simulink model "Relu_NoOutFB_4_4_1_HW_C6"  (R2012b)
settings: Solver=FixedStepDiscrete  SolverMode=SingleTasking  StartTime=0.0  StopTime=limSim  FixedStep=ts  RelTol=1e-3
undefined symbols (not defined in the file): alpha, delayMulx, delayMuly, delayROMSig, M2, M3, mu, ts
libraries: xbsIndex_r4 x1578, roblocks x1
(part 1 of 13)
settings Model: Creator=Marcelo  LastModifiedBy=snata
settings DataIOCC: SignalLoggingSaveFormat=ModelDataLogs
settings DebuggingCC: MultiTaskDSMMsg=warning  MultiTaskCondExecSysMsg=none  FcnCallInpInsideContextMsg=UseLocalSettings  StrictBusMsg=None
settings RTWCC: IncludeERTFirstTime=on
settings CodeAppCC: CustomSymbolStrType=$N$R$M_T  InternalIdentifier=Shortened
settings GRTTargetCC: CombineOutputUpdateFcns=off  GRTInterface=on

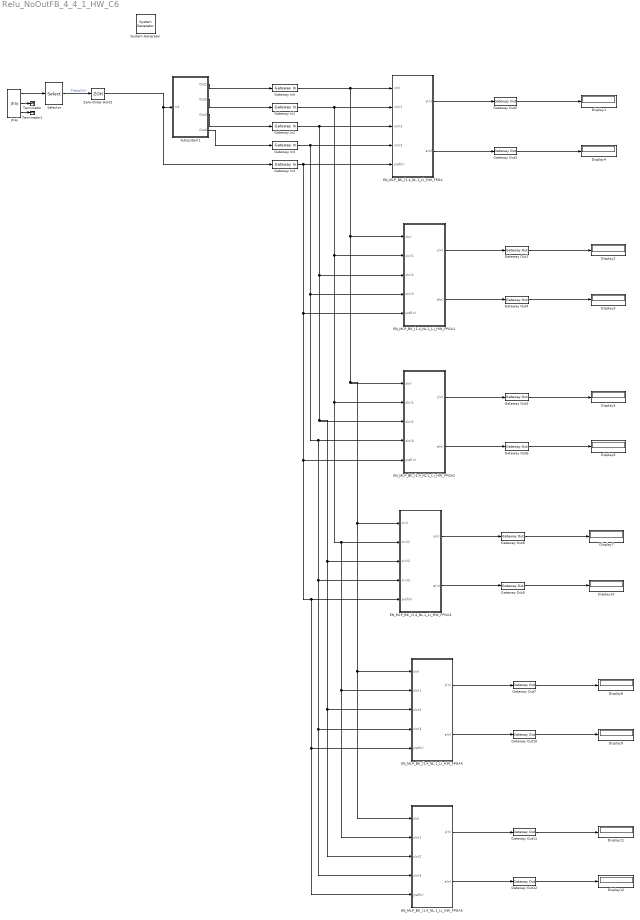
== system Relu_NoOutFB_4_4_1_HW_C6 ==
  " System Generator" : xbsIndex_r4/ System Generator  Tag=genX  xilinxfamily=virtex6  part=xc6vlx240t  speed=-1  package=ff1156  synthesis_tool=XST  clock_wrapper=Clock Enables  directory=C:/Users/snata/Documents/Netlists/RELU_SemReal_18_14  proj_type=Project Navigator  Synth_file=XST Defaults  Impl_file=ISE Defaults  testbench=off  simulink_period=0.01  sysclk_period=10  dcm_input_clock_period=10  incr_netlist=off  trim_vbits=Everywhere in SubSystem  dbl_ovrd=According to Block Masks  core_generation=According to Block Masks  run_coregen=off  deprecated_control=off  eval_field=0  block_type=sysgen
  Display{1..12} (12 alike) : Display
  EN_MLP_BK_(1,4_NL,1_L)_HW_FPGA : Subsystem
  EN_MLP_BK_(1,4_NL,1_L)_HW_FPGA1 : Subsystem
  EN_MLP_BK_(1,4_NL,1_L)_HW_FPGA2 : Subsystem
  EN_MLP_BK_(1,4_NL,1_L)_HW_FPGA3 : Subsystem
  EN_MLP_BK_(1,4_NL,1_L)_HW_FPGA4 : Subsystem
  EN_MLP_BK_(1,4_NL,1_L)_HW_FPGA5 : Subsystem
  Gateway In{1..5} (5 alike) : xbsIndex_r4/Gateway In  gui_display_data_type=Fixed-point  arith_type="Signed  (2's comp)"  n_bits=nb  bin_pt=bp  preci_type=Single  exp_width=8  frac_width=24  quantization="Round  (unbiased: +/- Inf)"  overflow=Saturate  period=ts  dbl_ovrd=off  timing_constraint=None  locs_specified=off  LOCs={}  UseAsADC=off  ADCChannel='1'  inherit_from_input=off  hdl_port=on  block_type=gatewayin
  Gateway Out{1..12} (12 alike) : xbsIndex_r4/Gateway Out  inherit_from_input=off  hdl_port=on  timing_constraint=None  locs_specified=off  LOCs={}  UseAsDAC=off  DACChannel='1'  block_type=gatewayout
      settings: infoedit="Gateway out block.  Converts Xilinx fixed point inputs into ouputs of type Simulink integer, double, or fixed point.<br><br>Hardware notes:  In hardware these blocks become top level output ports or are discarded, depending on how they are configured."
  Selector : Selector  InputPortWidth=3  IndexOptions=Index vector (dialog)  Indices=[1]  OutputSizes=1
  Subsystem1 : Subsystem
  Terminator : Terminator
  Terminator1 : Terminator
  Zero-Order Hold1 : ZeroOrderHold  SampleTime=ts
  jtraj : roblocks/Trajectory/jtraj  q0=[0 -pi/2 pi]  qf=[pi/2 pi/4 pi/2]  tmax=limSim  ts=ts
  wires:
  jtraj/1 -> Selector/1
  Subsystem1/1(Out1) -> Gateway In5/1
  Subsystem1/2(Out2) -> Gateway In1/1
  Subsystem1/3(Out3) -> Gateway In2/1
  Selector/1 -> Zero-Order Hold1/1  "Theta1(n)"
  Subsystem1/4(Out4) -> Gateway In3/1
  Zero-Order Hold1/1 -> Subsystem1/1(In1), Gateway In4/1
  jtraj/2 -> Terminator/1
  jtraj/3 -> Terminator1/1
  EN_MLP_BK_(1,4_NL,1_L)_HW_FPGA/2(e(n)) -> Gateway Out3/1
  Gateway Out3/1 -> Display4/1
  Gateway Out2/1 -> Display1/1
  EN_MLP_BK_(1,4_NL,1_L)_HW_FPGA/1(y(n)) -> Gateway Out2/1
  EN_MLP_BK_(1,4_NL,1_L)_HW_FPGA1/2(e(n)) -> Gateway Out4/1
  EN_MLP_BK_(1,4_NL,1_L)_HW_FPGA1/1(y(n)) -> Gateway Out1/1
  Gateway Out4/1 -> Display3/1
  Gateway Out1/1 -> Display2/1
  EN_MLP_BK_(1,4_NL,1_L)_HW_FPGA2/2(e(n)) -> Gateway Out6/1
  EN_MLP_BK_(1,4_NL,1_L)_HW_FPGA2/1(y(n)) -> Gateway Out5/1
  Gateway Out6/1 -> Display6/1
  Gateway Out5/1 -> Display5/1
  EN_MLP_BK_(1,4_NL,1_L)_HW_FPGA3/2(e(n)) -> Gateway Out9/1
  Gateway Out9/1 -> Display10/1
  Gateway Out8/1 -> Display7/1
  EN_MLP_BK_(1,4_NL,1_L)_HW_FPGA3/1(y(n)) -> Gateway Out8/1
  EN_MLP_BK_(1,4_NL,1_L)_HW_FPGA4/2(e(n)) -> Gateway Out10/1
  EN_MLP_BK_(1,4_NL,1_L)_HW_FPGA4/1(y(n)) -> Gateway Out7/1
  Gateway Out10/1 -> Display9/1
  Gateway Out7/1 -> Display8/1
  EN_MLP_BK_(1,4_NL,1_L)_HW_FPGA5/2(e(n)) -> Gateway Out12/1
  Gateway In5/1 -> EN_MLP_BK_(1,4_NL,1_L)_HW_FPGA3/1(x(n)), EN_MLP_BK_(1,4_NL,1_L)_HW_FPGA4/1(x(n)), EN_MLP_BK_(1,4_NL,1_L)_HW_FPGA5/1(x(n)), EN_MLP_BK_(1,4_NL,1_L)_HW_FPGA2/1(x(n)), EN_MLP_BK_(1,4_NL,1_L)_HW_FPGA1/1(x(n)), EN_MLP_BK_(1,4_NL,1_L)_HW_FPGA/1(x(n))
  Gateway In4/1 -> EN_MLP_BK_(1,4_NL,1_L)_HW_FPGA3/5(yref(n)), EN_MLP_BK_(1,4_NL,1_L)_HW_FPGA4/5(yref(n)), EN_MLP_BK_(1,4_NL,1_L)_HW_FPGA5/5(yref(n)), EN_MLP_BK_(1,4_NL,1_L)_HW_FPGA2/5(yref(n)), EN_MLP_BK_(1,4_NL,1_L)_HW_FPGA1/5(yref(n)), EN_MLP_BK_(1,4_NL,1_L)_HW_FPGA/5(yref(n))
  Gateway In1/1 -> EN_MLP_BK_(1,4_NL,1_L)_HW_FPGA3/2(x(n)1), EN_MLP_BK_(1,4_NL,1_L)_HW_FPGA4/2(x(n)1), EN_MLP_BK_(1,4_NL,1_L)_HW_FPGA5/2(x(n)1), EN_MLP_BK_(1,4_NL,1_L)_HW_FPGA2/2(x(n)1), EN_MLP_BK_(1,4_NL,1_L)_HW_FPGA1/2(x(n)1), EN_MLP_BK_(1,4_NL,1_L)_HW_FPGA/2(x(n)1)
  Gateway In2/1 -> EN_MLP_BK_(1,4_NL,1_L)_HW_FPGA3/3(x(n)2), EN_MLP_BK_(1,4_NL,1_L)_HW_FPGA4/3(x(n)2), EN_MLP_BK_(1,4_NL,1_L)_HW_FPGA5/3(x(n)2), EN_MLP_BK_(1,4_NL,1_L)_HW_FPGA2/3(x(n)2), EN_MLP_BK_(1,4_NL,1_L)_HW_FPGA1/3(x(n)2), EN_MLP_BK_(1,4_NL,1_L)_HW_FPGA/3(x(n)2)
  EN_MLP_BK_(1,4_NL,1_L)_HW_FPGA5/1(y(n)) -> Gateway Out11/1
  Gateway In3/1 -> EN_MLP_BK_(1,4_NL,1_L)_HW_FPGA3/4(x(n)3), EN_MLP_BK_(1,4_NL,1_L)_HW_FPGA4/4(x(n)3), EN_MLP_BK_(1,4_NL,1_L)_HW_FPGA5/4(x(n)3), EN_MLP_BK_(1,4_NL,1_L)_HW_FPGA2/4(x(n)3), EN_MLP_BK_(1,4_NL,1_L)_HW_FPGA1/4(x(n)3), EN_MLP_BK_(1,4_NL,1_L)_HW_FPGA/4(x(n)3)
  Gateway Out12/1 -> Display12/1
  Gateway Out11/1 -> Display11/1

== system Relu_NoOutFB_4_4_1_HW_C6/EN_MLP_BK_(1,4_NL,1_L)_HW_FPGA ==
  x(n) : Inport
  x(n)1 : Inport  Port=2
  x(n)2 : Inport  Port=3
  x(n)3 : Inport  Port=4
  yref(n) : Inport  Port=5
  MLP_BK_(2,4_NL,1_L)_HW_FPGA : Subsystem
  y(n) : Outport
  e(n) : Outport  Port=2
  wires:
  yref(n)/1 -> MLP_BK_(2,4_NL,1_L)_HW_FPGA/5(y_ref(n))
  x(n)/1 -> MLP_BK_(2,4_NL,1_L)_HW_FPGA/1(x_1(n))  "x(n)"
  MLP_BK_(2,4_NL,1_L)_HW_FPGA/2(e(n)) -> e(n)/1
  x(n)1/1 -> MLP_BK_(2,4_NL,1_L)_HW_FPGA/2(x_2(n))
  x(n)2/1 -> MLP_BK_(2,4_NL,1_L)_HW_FPGA/3(x_3(n))
  MLP_BK_(2,4_NL,1_L)_HW_FPGA/1(y(n)) -> y(n)/1
  x(n)3/1 -> MLP_BK_(2,4_NL,1_L)_HW_FPGA/4(x_4(n))

== system Relu_NoOutFB_4_4_1_HW_C6/EN_MLP_BK_(1,4_NL,1_L)_HW_FPGA1 ==
  x(n) : Inport
  x(n)1 : Inport  Port=2
  x(n)2 : Inport  Port=3
  x(n)3 : Inport  Port=4
  yref(n) : Inport  Port=5
  MLP_BK_(2,4_NL,1_L)_HW_FPGA : Subsystem
  y(n) : Outport
  e(n) : Outport  Port=2
  wires:
  x(n)3/1 -> MLP_BK_(2,4_NL,1_L)_HW_FPGA/4(x_4(n))
  MLP_BK_(2,4_NL,1_L)_HW_FPGA/1(y(n)) -> y(n)/1
  x(n)2/1 -> MLP_BK_(2,4_NL,1_L)_HW_FPGA/3(x_3(n))
  x(n)1/1 -> MLP_BK_(2,4_NL,1_L)_HW_FPGA/2(x_2(n))
  MLP_BK_(2,4_NL,1_L)_HW_FPGA/2(e(n)) -> e(n)/1
  x(n)/1 -> MLP_BK_(2,4_NL,1_L)_HW_FPGA/1(x_1(n))  "x(n)"
  yref(n)/1 -> MLP_BK_(2,4_NL,1_L)_HW_FPGA/5(y_ref(n))

== system Relu_NoOutFB_4_4_1_HW_C6/EN_MLP_BK_(1,4_NL,1_L)_HW_FPGA2 ==
  x(n) : Inport
  x(n)1 : Inport  Port=2
  x(n)2 : Inport  Port=3
  x(n)3 : Inport  Port=4
  yref(n) : Inport  Port=5
  MLP_BK_(2,4_NL,1_L)_HW_FPGA : Subsystem
  y(n) : Outport
  e(n) : Outport  Port=2
  wires:
  yref(n)/1 -> MLP_BK_(2,4_NL,1_L)_HW_FPGA/5(y_ref(n))
  x(n)/1 -> MLP_BK_(2,4_NL,1_L)_HW_FPGA/1(x_1(n))  "x(n)"
  MLP_BK_(2,4_NL,1_L)_HW_FPGA/2(e(n)) -> e(n)/1
  x(n)1/1 -> MLP_BK_(2,4_NL,1_L)_HW_FPGA/2(x_2(n))
  x(n)2/1 -> MLP_BK_(2,4_NL,1_L)_HW_FPGA/3(x_3(n))
  MLP_BK_(2,4_NL,1_L)_HW_FPGA/1(y(n)) -> y(n)/1
  x(n)3/1 -> MLP_BK_(2,4_NL,1_L)_HW_FPGA/4(x_4(n))

== system Relu_NoOutFB_4_4_1_HW_C6/EN_MLP_BK_(1,4_NL,1_L)_HW_FPGA3 ==
  x(n) : Inport
  x(n)1 : Inport  Port=2
  x(n)2 : Inport  Port=3
  x(n)3 : Inport  Port=4
  yref(n) : Inport  Port=5
  MLP_BK_(2,4_NL,1_L)_HW_FPGA : Subsystem
  y(n) : Outport
  e(n) : Outport  Port=2
  wires:
  x(n)3/1 -> MLP_BK_(2,4_NL,1_L)_HW_FPGA/4(x_4(n))
  MLP_BK_(2,4_NL,1_L)_HW_FPGA/1(y(n)) -> y(n)/1
  x(n)2/1 -> MLP_BK_(2,4_NL,1_L)_HW_FPGA/3(x_3(n))
  x(n)1/1 -> MLP_BK_(2,4_NL,1_L)_HW_FPGA/2(x_2(n))
  MLP_BK_(2,4_NL,1_L)_HW_FPGA/2(e(n)) -> e(n)/1
  x(n)/1 -> MLP_BK_(2,4_NL,1_L)_HW_FPGA/1(x_1(n))  "x(n)"
  yref(n)/1 -> MLP_BK_(2,4_NL,1_L)_HW_FPGA/5(y_ref(n))

== system Relu_NoOutFB_4_4_1_HW_C6/EN_MLP_BK_(1,4_NL,1_L)_HW_FPGA4 ==
  x(n) : Inport
  x(n)1 : Inport  Port=2
  x(n)2 : Inport  Port=3
  x(n)3 : Inport  Port=4
  yref(n) : Inport  Port=5
  MLP_BK_(2,4_NL,1_L)_HW_FPGA : Subsystem
  y(n) : Outport
  e(n) : Outport  Port=2
  wires:
  yref(n)/1 -> MLP_BK_(2,4_NL,1_L)_HW_FPGA/5(y_ref(n))
  x(n)/1 -> MLP_BK_(2,4_NL,1_L)_HW_FPGA/1(x_1(n))  "x(n)"
  MLP_BK_(2,4_NL,1_L)_HW_FPGA/2(e(n)) -> e(n)/1
  x(n)1/1 -> MLP_BK_(2,4_NL,1_L)_HW_FPGA/2(x_2(n))
  x(n)2/1 -> MLP_BK_(2,4_NL,1_L)_HW_FPGA/3(x_3(n))
  MLP_BK_(2,4_NL,1_L)_HW_FPGA/1(y(n)) -> y(n)/1
  x(n)3/1 -> MLP_BK_(2,4_NL,1_L)_HW_FPGA/4(x_4(n))

== system Relu_NoOutFB_4_4_1_HW_C6/EN_MLP_BK_(1,4_NL,1_L)_HW_FPGA5 ==
  x(n) : Inport
  x(n)1 : Inport  Port=2
  x(n)2 : Inport  Port=3
  x(n)3 : Inport  Port=4
  yref(n) : Inport  Port=5
  MLP_BK_(2,4_NL,1_L)_HW_FPGA : Subsystem
  y(n) : Outport
  e(n) : Outport  Port=2
  wires:
  x(n)3/1 -> MLP_BK_(2,4_NL,1_L)_HW_FPGA/4(x_4(n))
  MLP_BK_(2,4_NL,1_L)_HW_FPGA/1(y(n)) -> y(n)/1
  x(n)2/1 -> MLP_BK_(2,4_NL,1_L)_HW_FPGA/3(x_3(n))
  x(n)1/1 -> MLP_BK_(2,4_NL,1_L)_HW_FPGA/2(x_2(n))
  MLP_BK_(2,4_NL,1_L)_HW_FPGA/2(e(n)) -> e(n)/1
  x(n)/1 -> MLP_BK_(2,4_NL,1_L)_HW_FPGA/1(x_1(n))  "x(n)"
  yref(n)/1 -> MLP_BK_(2,4_NL,1_L)_HW_FPGA/5(y_ref(n))

== system Relu_NoOutFB_4_4_1_HW_C6/Subsystem1 ==
  In1 : Inport
  Delay{1..6} (6 alike) : Delay  DelayLength=1
  Terminator : Terminator
  Out1 : Outport
  Out2 : Outport  Port=2
  Out3 : Outport  Port=3
  Out4 : Outport  Port=4
  wires:
  Delay4/1 -> Delay1/1, Out3/1
  Delay2/1 -> Out2/1, Delay4/1
  Delay3/1 -> Out1/1, Delay2/1
  In1/1 -> Delay3/1
  Delay1/1 -> Out4/1, Delay5/1
  Delay5/1 -> Delay6/1
  Delay6/1 -> Terminator/1

== system Relu_NoOutFB_4_4_1_HW_C6/EN_MLP_BK_(1,4_NL,1_L)_HW_FPGA/MLP_BK_(2,4_NL,1_L)_HW_FPGA ==
  x_1(n) : Inport
  x_2(n) : Inport  Port=2
  x_3(n) : Inport  Port=3
  x_4(n) : Inport  Port=4
  y_ref(n) : Inport  Port=5
  AddSub : xbsIndex_r4/AddSub  mode=Subtraction  use_carryin=off  use_carryout=off  en=off  latency=0  precision=User Defined  arith_type="Signed  (2's comp)"  n_bits=nb  bin_pt=bp  quantization="Round  (unbiased: +/- Inf)"  overflow=Wrap  dbl_ovrd=off  use_behavioral_HDL=off  hw_selection=Fabric  pipelined=off  block_type=addsub
  BK (2,4_NL,1_L) : Subsystem
  Delay{,1..4} (5 alike) : xbsIndex_r4/Delay  rst=off  infoeditControl=Selection of Reset will increase slice count due to use of real FFs and instead of SRLs  en=off  latency=delayROMSig+delayMulx+delayMuly  dbl_ovrd=off  reg_retiming=off  block_type=delay
  MLP (2,4_NL,1_L) : Subsystem
  y(n) : Outport
  e(n) : Outport  Port=2
  wires:
  Delay/1 -> AddSub/1
  y_ref(n)/1 -> Delay/1
  x_1(n)/1 -> MLP (2,4_NL,1_L)/4(x_1(n))
  BK (2,4_NL,1_L)/1(Wy_10(n)) -> MLP (2,4_NL,1_L)/29(Wy_10(n))
  AddSub/1 -> e(n)/1, BK (2,4_NL,1_L)/11(e(n))
  BK (2,4_NL,1_L)/2(Wy_11(n)) -> MLP (2,4_NL,1_L)/28(Wy_11(n))
  x_2(n)/1 -> MLP (2,4_NL,1_L)/3(x_2(n))
  x_3(n)/1 -> MLP (2,4_NL,1_L)/2(x_3(n))
  x_4(n)/1 -> MLP (2,4_NL,1_L)/1(x_4(n))
  BK (2,4_NL,1_L)/3(Wy_12(n)) -> MLP (2,4_NL,1_L)/27(Wy_12(n))
  BK (2,4_NL,1_L)/4(Wy_13(n)) -> MLP (2,4_NL,1_L)/26(Wy_13(n))
  BK (2,4_NL,1_L)/5(Wy_14(n)) -> MLP (2,4_NL,1_L)/25(Wy_14(n))
  BK (2,4_NL,1_L)/6(Wx_10(n)) -> MLP (2,4_NL,1_L)/24(Wx_10(n))
  BK (2,4_NL,1_L)/7(Wx_11(n)) -> MLP (2,4_NL,1_L)/23(Wx_11(n))
  BK (2,4_NL,1_L)/8(Wx_12(n)) -> MLP (2,4_NL,1_L)/22(Wx_12(n))
  BK (2,4_NL,1_L)/9(Wx_13(n)) -> MLP (2,4_NL,1_L)/21(Wx_13(n))
  BK (2,4_NL,1_L)/10(Wx_14(n)) -> MLP (2,4_NL,1_L)/20(Wx_14(n))
  BK (2,4_NL,1_L)/11(Wx_20(n)) -> MLP (2,4_NL,1_L)/19(Wx_20(n))
  BK (2,4_NL,1_L)/12(Wx_21(n)) -> MLP (2,4_NL,1_L)/18(Wx_21(n))
  BK (2,4_NL,1_L)/13(Wx_22(n)) -> MLP (2,4_NL,1_L)/17(Wx_22(n))
  BK (2,4_NL,1_L)/14(Wx_23(n)) -> MLP (2,4_NL,1_L)/16(Wx_23(n))
  BK (2,4_NL,1_L)/15(Wx_24(n)) -> MLP (2,4_NL,1_L)/15(Wx_24(n))
  BK (2,4_NL,1_L)/16(Wx_30(n)) -> MLP (2,4_NL,1_L)/14(Wx_30(n))
  BK (2,4_NL,1_L)/17(Wx_31(n)) -> MLP (2,4_NL,1_L)/13(Wx_31(n))
  BK (2,4_NL,1_L)/18(Wx_32(n)) -> MLP (2,4_NL,1_L)/12(Wx_32(n)1)
  BK (2,4_NL,1_L)/19(Wx_33(n)) -> MLP (2,4_NL,1_L)/11(Wx_33(n))
  BK (2,4_NL,1_L)/20(Wx_34(n)) -> MLP (2,4_NL,1_L)/10(Wx_34(n))
  BK (2,4_NL,1_L)/21(Wx_40(n)) -> MLP (2,4_NL,1_L)/9(Wx_40(n))
  BK (2,4_NL,1_L)/22(Wx_41(n)) -> MLP (2,4_NL,1_L)/8(Wx_41(n))
  BK (2,4_NL,1_L)/23(Wx_42(n)) -> MLP (2,4_NL,1_L)/7(Wx_42(n))
  BK (2,4_NL,1_L)/24(Wx_43(n)) -> MLP (2,4_NL,1_L)/6(Wx_43(n))
  BK (2,4_NL,1_L)/25(Wx_44(n)) -> MLP (2,4_NL,1_L)/5(Wx_44(n))
  MLP (2,4_NL,1_L)/11(x_4(n)bp) -> Delay1/1
  MLP (2,4_NL,1_L)/10(x_3(n)bp) -> Delay2/1
  MLP (2,4_NL,1_L)/9(x_2(n)bp) -> Delay3/1
  MLP (2,4_NL,1_L)/8(x_1(n)bp) -> Delay4/1
  MLP (2,4_NL,1_L)/6(z_4(n)) -> BK (2,4_NL,1_L)/6(z_4(n))
  MLP (2,4_NL,1_L)/5(z_3(n)) -> BK (2,4_NL,1_L)/7(z_3(n))
  MLP (2,4_NL,1_L)/4(z_2(n)) -> BK (2,4_NL,1_L)/8(z_2(n))
  MLP (2,4_NL,1_L)/3(z_1(n)) -> BK (2,4_NL,1_L)/9(z_1(n))
  MLP (2,4_NL,1_L)/2(z_0(n)) -> BK (2,4_NL,1_L)/10(z_0(n))
  MLP (2,4_NL,1_L)/1(y_0(n)) -> y(n)/1, AddSub/2
  Delay1/1 -> BK (2,4_NL,1_L)/1(x_4(n))
  Delay2/1 -> BK (2,4_NL,1_L)/2(x_3(n))
  Delay3/1 -> BK (2,4_NL,1_L)/3(x_2(n))
  Delay4/1 -> BK (2,4_NL,1_L)/4(x_1(n))
  MLP (2,4_NL,1_L)/7(x_0(n)bp) -> BK (2,4_NL,1_L)/5(x_0(n))

== system Relu_NoOutFB_4_4_1_HW_C6/EN_MLP_BK_(1,4_NL,1_L)_HW_FPGA1/MLP_BK_(2,4_NL,1_L)_HW_FPGA ==
  x_1(n) : Inport
  x_2(n) : Inport  Port=2
  x_3(n) : Inport  Port=3
  x_4(n) : Inport  Port=4
  y_ref(n) : Inport  Port=5
  AddSub : xbsIndex_r4/AddSub  mode=Subtraction  use_carryin=off  use_carryout=off  en=off  latency=0  precision=User Defined  arith_type="Signed  (2's comp)"  n_bits=nb  bin_pt=bp  quantization="Round  (unbiased: +/- Inf)"  overflow=Wrap  dbl_ovrd=off  use_behavioral_HDL=off  hw_selection=Fabric  pipelined=off  block_type=addsub
  BK (2,4_NL,1_L) : Subsystem
  Delay{,1..4} (5 alike) : xbsIndex_r4/Delay  rst=off  infoeditControl=Selection of Reset will increase slice count due to use of real FFs and instead of SRLs  en=off  latency=delayROMSig+delayMulx+delayMuly  dbl_ovrd=off  reg_retiming=off  block_type=delay
  MLP (2,4_NL,1_L) : Subsystem
  y(n) : Outport
  e(n) : Outport  Port=2
  wires:
  MLP (2,4_NL,1_L)/7(x_0(n)bp) -> BK (2,4_NL,1_L)/5(x_0(n))
  Delay4/1 -> BK (2,4_NL,1_L)/4(x_1(n))
  Delay3/1 -> BK (2,4_NL,1_L)/3(x_2(n))
  Delay2/1 -> BK (2,4_NL,1_L)/2(x_3(n))
  Delay1/1 -> BK (2,4_NL,1_L)/1(x_4(n))
  MLP (2,4_NL,1_L)/1(y_0(n)) -> AddSub/2, y(n)/1
  MLP (2,4_NL,1_L)/2(z_0(n)) -> BK (2,4_NL,1_L)/10(z_0(n))
  MLP (2,4_NL,1_L)/3(z_1(n)) -> BK (2,4_NL,1_L)/9(z_1(n))
  MLP (2,4_NL,1_L)/4(z_2(n)) -> BK (2,4_NL,1_L)/8(z_2(n))
  MLP (2,4_NL,1_L)/5(z_3(n)) -> BK (2,4_NL,1_L)/7(z_3(n))
  MLP (2,4_NL,1_L)/6(z_4(n)) -> BK (2,4_NL,1_L)/6(z_4(n))
  MLP (2,4_NL,1_L)/8(x_1(n)bp) -> Delay4/1
  MLP (2,4_NL,1_L)/9(x_2(n)bp) -> Delay3/1
  MLP (2,4_NL,1_L)/10(x_3(n)bp) -> Delay2/1
  MLP (2,4_NL,1_L)/11(x_4(n)bp) -> Delay1/1
  BK (2,4_NL,1_L)/25(Wx_44(n)) -> MLP (2,4_NL,1_L)/5(Wx_44(n))
  BK (2,4_NL,1_L)/24(Wx_43(n)) -> MLP (2,4_NL,1_L)/6(Wx_43(n))
  BK (2,4_NL,1_L)/23(Wx_42(n)) -> MLP (2,4_NL,1_L)/7(Wx_42(n))
  BK (2,4_NL,1_L)/22(Wx_41(n)) -> MLP (2,4_NL,1_L)/8(Wx_41(n))
  BK (2,4_NL,1_L)/21(Wx_40(n)) -> MLP (2,4_NL,1_L)/9(Wx_40(n))
  BK (2,4_NL,1_L)/20(Wx_34(n)) -> MLP (2,4_NL,1_L)/10(Wx_34(n))
  BK (2,4_NL,1_L)/19(Wx_33(n)) -> MLP (2,4_NL,1_L)/11(Wx_33(n))
  BK (2,4_NL,1_L)/18(Wx_32(n)) -> MLP (2,4_NL,1_L)/12(Wx_32(n)1)
  BK (2,4_NL,1_L)/17(Wx_31(n)) -> MLP (2,4_NL,1_L)/13(Wx_31(n))
  BK (2,4_NL,1_L)/16(Wx_30(n)) -> MLP (2,4_NL,1_L)/14(Wx_30(n))
  BK (2,4_NL,1_L)/15(Wx_24(n)) -> MLP (2,4_NL,1_L)/15(Wx_24(n))
  BK (2,4_NL,1_L)/14(Wx_23(n)) -> MLP (2,4_NL,1_L)/16(Wx_23(n))
  BK (2,4_NL,1_L)/13(Wx_22(n)) -> MLP (2,4_NL,1_L)/17(Wx_22(n))
  BK (2,4_NL,1_L)/12(Wx_21(n)) -> MLP (2,4_NL,1_L)/18(Wx_21(n))
  BK (2,4_NL,1_L)/11(Wx_20(n)) -> MLP (2,4_NL,1_L)/19(Wx_20(n))
  BK (2,4_NL,1_L)/10(Wx_14(n)) -> MLP (2,4_NL,1_L)/20(Wx_14(n))
  BK (2,4_NL,1_L)/9(Wx_13(n)) -> MLP (2,4_NL,1_L)/21(Wx_13(n))
  BK (2,4_NL,1_L)/8(Wx_12(n)) -> MLP (2,4_NL,1_L)/22(Wx_12(n))
  BK (2,4_NL,1_L)/7(Wx_11(n)) -> MLP (2,4_NL,1_L)/23(Wx_11(n))
  BK (2,4_NL,1_L)/6(Wx_10(n)) -> MLP (2,4_NL,1_L)/24(Wx_10(n))
  BK (2,4_NL,1_L)/5(Wy_14(n)) -> MLP (2,4_NL,1_L)/25(Wy_14(n))
  BK (2,4_NL,1_L)/4(Wy_13(n)) -> MLP (2,4_NL,1_L)/26(Wy_13(n))
  BK (2,4_NL,1_L)/3(Wy_12(n)) -> MLP (2,4_NL,1_L)/27(Wy_12(n))
  x_4(n)/1 -> MLP (2,4_NL,1_L)/1(x_4(n))
  x_3(n)/1 -> MLP (2,4_NL,1_L)/2(x_3(n))
  x_2(n)/1 -> MLP (2,4_NL,1_L)/3(x_2(n))
  BK (2,4_NL,1_L)/2(Wy_11(n)) -> MLP (2,4_NL,1_L)/28(Wy_11(n))
  AddSub/1 -> BK (2,4_NL,1_L)/11(e(n)), e(n)/1
  BK (2,4_NL,1_L)/1(Wy_10(n)) -> MLP (2,4_NL,1_L)/29(Wy_10(n))
  x_1(n)/1 -> MLP (2,4_NL,1_L)/4(x_1(n))
  y_ref(n)/1 -> Delay/1
  Delay/1 -> AddSub/1

== system Relu_NoOutFB_4_4_1_HW_C6/EN_MLP_BK_(1,4_NL,1_L)_HW_FPGA2/MLP_BK_(2,4_NL,1_L)_HW_FPGA ==
  x_1(n) : Inport
  x_2(n) : Inport  Port=2
  x_3(n) : Inport  Port=3
  x_4(n) : Inport  Port=4
  y_ref(n) : Inport  Port=5
  AddSub : xbsIndex_r4/AddSub  mode=Subtraction  use_carryin=off  use_carryout=off  en=off  latency=0  precision=User Defined  arith_type="Signed  (2's comp)"  n_bits=nb  bin_pt=bp  quantization="Round  (unbiased: +/- Inf)"  overflow=Wrap  dbl_ovrd=off  use_behavioral_HDL=off  hw_selection=Fabric  pipelined=off  block_type=addsub
  BK (2,4_NL,1_L) : Subsystem
  Delay{,1..4} (5 alike) : xbsIndex_r4/Delay  rst=off  infoeditControl=Selection of Reset will increase slice count due to use of real FFs and instead of SRLs  en=off  latency=delayROMSig+delayMulx+delayMuly  dbl_ovrd=off  reg_retiming=off  block_type=delay
  MLP (2,4_NL,1_L) : Subsystem
  y(n) : Outport
  e(n) : Outport  Port=2
  wires:
  Delay/1 -> AddSub/1
  y_ref(n)/1 -> Delay/1
  x_1(n)/1 -> MLP (2,4_NL,1_L)/4(x_1(n))
  BK (2,4_NL,1_L)/1(Wy_10(n)) -> MLP (2,4_NL,1_L)/29(Wy_10(n))
  AddSub/1 -> e(n)/1, BK (2,4_NL,1_L)/11(e(n))
  BK (2,4_NL,1_L)/2(Wy_11(n)) -> MLP (2,4_NL,1_L)/28(Wy_11(n))
  x_2(n)/1 -> MLP (2,4_NL,1_L)/3(x_2(n))
  x_3(n)/1 -> MLP (2,4_NL,1_L)/2(x_3(n))
  x_4(n)/1 -> MLP (2,4_NL,1_L)/1(x_4(n))
  BK (2,4_NL,1_L)/3(Wy_12(n)) -> MLP (2,4_NL,1_L)/27(Wy_12(n))
  BK (2,4_NL,1_L)/4(Wy_13(n)) -> MLP (2,4_NL,1_L)/26(Wy_13(n))
  BK (2,4_NL,1_L)/5(Wy_14(n)) -> MLP (2,4_NL,1_L)/25(Wy_14(n))
  BK (2,4_NL,1_L)/6(Wx_10(n)) -> MLP (2,4_NL,1_L)/24(Wx_10(n))
  BK (2,4_NL,1_L)/7(Wx_11(n)) -> MLP (2,4_NL,1_L)/23(Wx_11(n))
  BK (2,4_NL,1_L)/8(Wx_12(n)) -> MLP (2,4_NL,1_L)/22(Wx_12(n))
  BK (2,4_NL,1_L)/9(Wx_13(n)) -> MLP (2,4_NL,1_L)/21(Wx_13(n))
  BK (2,4_NL,1_L)/10(Wx_14(n)) -> MLP (2,4_NL,1_L)/20(Wx_14(n))
  BK (2,4_NL,1_L)/11(Wx_20(n)) -> MLP (2,4_NL,1_L)/19(Wx_20(n))
  BK (2,4_NL,1_L)/12(Wx_21(n)) -> MLP (2,4_NL,1_L)/18(Wx_21(n))
  BK (2,4_NL,1_L)/13(Wx_22(n)) -> MLP (2,4_NL,1_L)/17(Wx_22(n))
  BK (2,4_NL,1_L)/14(Wx_23(n)) -> MLP (2,4_NL,1_L)/16(Wx_23(n))
  BK (2,4_NL,1_L)/15(Wx_24(n)) -> MLP (2,4_NL,1_L)/15(Wx_24(n))
  BK (2,4_NL,1_L)/16(Wx_30(n)) -> MLP (2,4_NL,1_L)/14(Wx_30(n))
  BK (2,4_NL,1_L)/17(Wx_31(n)) -> MLP (2,4_NL,1_L)/13(Wx_31(n))
  BK (2,4_NL,1_L)/18(Wx_32(n)) -> MLP (2,4_NL,1_L)/12(Wx_32(n)1)
  BK (2,4_NL,1_L)/19(Wx_33(n)) -> MLP (2,4_NL,1_L)/11(Wx_33(n))
  BK (2,4_NL,1_L)/20(Wx_34(n)) -> MLP (2,4_NL,1_L)/10(Wx_34(n))
  BK (2,4_NL,1_L)/21(Wx_40(n)) -> MLP (2,4_NL,1_L)/9(Wx_40(n))
  BK (2,4_NL,1_L)/22(Wx_41(n)) -> MLP (2,4_NL,1_L)/8(Wx_41(n))
  BK (2,4_NL,1_L)/23(Wx_42(n)) -> MLP (2,4_NL,1_L)/7(Wx_42(n))
  BK (2,4_NL,1_L)/24(Wx_43(n)) -> MLP (2,4_NL,1_L)/6(Wx_43(n))
  BK (2,4_NL,1_L)/25(Wx_44(n)) -> MLP (2,4_NL,1_L)/5(Wx_44(n))
  MLP (2,4_NL,1_L)/11(x_4(n)bp) -> Delay1/1
  MLP (2,4_NL,1_L)/10(x_3(n)bp) -> Delay2/1
  MLP (2,4_NL,1_L)/9(x_2(n)bp) -> Delay3/1
  MLP (2,4_NL,1_L)/8(x_1(n)bp) -> Delay4/1
  MLP (2,4_NL,1_L)/6(z_4(n)) -> BK (2,4_NL,1_L)/6(z_4(n))
  MLP (2,4_NL,1_L)/5(z_3(n)) -> BK (2,4_NL,1_L)/7(z_3(n))
  MLP (2,4_NL,1_L)/4(z_2(n)) -> BK (2,4_NL,1_L)/8(z_2(n))
  MLP (2,4_NL,1_L)/3(z_1(n)) -> BK (2,4_NL,1_L)/9(z_1(n))
  MLP (2,4_NL,1_L)/2(z_0(n)) -> BK (2,4_NL,1_L)/10(z_0(n))
  MLP (2,4_NL,1_L)/1(y_0(n)) -> y(n)/1, AddSub/2
  Delay1/1 -> BK (2,4_NL,1_L)/1(x_4(n))
  Delay2/1 -> BK (2,4_NL,1_L)/2(x_3(n))
  Delay3/1 -> BK (2,4_NL,1_L)/3(x_2(n))
  Delay4/1 -> BK (2,4_NL,1_L)/4(x_1(n))
  MLP (2,4_NL,1_L)/7(x_0(n)bp) -> BK (2,4_NL,1_L)/5(x_0(n))

== system Relu_NoOutFB_4_4_1_HW_C6/EN_MLP_BK_(1,4_NL,1_L)_HW_FPGA3/MLP_BK_(2,4_NL,1_L)_HW_FPGA ==
  x_1(n) : Inport
  x_2(n) : Inport  Port=2
  x_3(n) : Inport  Port=3
  x_4(n) : Inport  Port=4
  y_ref(n) : Inport  Port=5
  AddSub : xbsIndex_r4/AddSub  mode=Subtraction  use_carryin=off  use_carryout=off  en=off  latency=0  precision=User Defined  arith_type="Signed  (2's comp)"  n_bits=nb  bin_pt=bp  quantization="Round  (unbiased: +/- Inf)"  overflow=Wrap  dbl_ovrd=off  use_behavioral_HDL=off  hw_selection=Fabric  pipelined=off  block_type=addsub
  BK (2,4_NL,1_L) : Subsystem
  Delay{,1..4} (5 alike) : xbsIndex_r4/Delay  rst=off  infoeditControl=Selection of Reset will increase slice count due to use of real FFs and instead of SRLs  en=off  latency=delayROMSig+delayMulx+delayMuly  dbl_ovrd=off  reg_retiming=off  block_type=delay
  MLP (2,4_NL,1_L) : Subsystem
  y(n) : Outport
  e(n) : Outport  Port=2
  wires:
  MLP (2,4_NL,1_L)/7(x_0(n)bp) -> BK (2,4_NL,1_L)/5(x_0(n))
  Delay4/1 -> BK (2,4_NL,1_L)/4(x_1(n))
  Delay3/1 -> BK (2,4_NL,1_L)/3(x_2(n))
  Delay2/1 -> BK (2,4_NL,1_L)/2(x_3(n))
  Delay1/1 -> BK (2,4_NL,1_L)/1(x_4(n))
  MLP (2,4_NL,1_L)/1(y_0(n)) -> AddSub/2, y(n)/1
  MLP (2,4_NL,1_L)/2(z_0(n)) -> BK (2,4_NL,1_L)/10(z_0(n))
  MLP (2,4_NL,1_L)/3(z_1(n)) -> BK (2,4_NL,1_L)/9(z_1(n))
  MLP (2,4_NL,1_L)/4(z_2(n)) -> BK (2,4_NL,1_L)/8(z_2(n))
  MLP (2,4_NL,1_L)/5(z_3(n)) -> BK (2,4_NL,1_L)/7(z_3(n))
  MLP (2,4_NL,1_L)/6(z_4(n)) -> BK (2,4_NL,1_L)/6(z_4(n))
  MLP (2,4_NL,1_L)/8(x_1(n)bp) -> Delay4/1
  MLP (2,4_NL,1_L)/9(x_2(n)bp) -> Delay3/1
  MLP (2,4_NL,1_L)/10(x_3(n)bp) -> Delay2/1
  MLP (2,4_NL,1_L)/11(x_4(n)bp) -> Delay1/1
  BK (2,4_NL,1_L)/25(Wx_44(n)) -> MLP (2,4_NL,1_L)/5(Wx_44(n))
  BK (2,4_NL,1_L)/24(Wx_43(n)) -> MLP (2,4_NL,1_L)/6(Wx_43(n))
  BK (2,4_NL,1_L)/23(Wx_42(n)) -> MLP (2,4_NL,1_L)/7(Wx_42(n))
  BK (2,4_NL,1_L)/22(Wx_41(n)) -> MLP (2,4_NL,1_L)/8(Wx_41(n))
  BK (2,4_NL,1_L)/21(Wx_40(n)) -> MLP (2,4_NL,1_L)/9(Wx_40(n))
  BK (2,4_NL,1_L)/20(Wx_34(n)) -> MLP (2,4_NL,1_L)/10(Wx_34(n))
  BK (2,4_NL,1_L)/19(Wx_33(n)) -> MLP (2,4_NL,1_L)/11(Wx_33(n))
  BK (2,4_NL,1_L)/18(Wx_32(n)) -> MLP (2,4_NL,1_L)/12(Wx_32(n)1)
  BK (2,4_NL,1_L)/17(Wx_31(n)) -> MLP (2,4_NL,1_L)/13(Wx_31(n))
  BK (2,4_NL,1_L)/16(Wx_30(n)) -> MLP (2,4_NL,1_L)/14(Wx_30(n))
  BK (2,4_NL,1_L)/15(Wx_24(n)) -> MLP (2,4_NL,1_L)/15(Wx_24(n))
  BK (2,4_NL,1_L)/14(Wx_23(n)) -> MLP (2,4_NL,1_L)/16(Wx_23(n))
  BK (2,4_NL,1_L)/13(Wx_22(n)) -> MLP (2,4_NL,1_L)/17(Wx_22(n))
  BK (2,4_NL,1_L)/12(Wx_21(n)) -> MLP (2,4_NL,1_L)/18(Wx_21(n))
  BK (2,4_NL,1_L)/11(Wx_20(n)) -> MLP (2,4_NL,1_L)/19(Wx_20(n))
  BK (2,4_NL,1_L)/10(Wx_14(n)) -> MLP (2,4_NL,1_L)/20(Wx_14(n))
  BK (2,4_NL,1_L)/9(Wx_13(n)) -> MLP (2,4_NL,1_L)/21(Wx_13(n))
  BK (2,4_NL,1_L)/8(Wx_12(n)) -> MLP (2,4_NL,1_L)/22(Wx_12(n))
  BK (2,4_NL,1_L)/7(Wx_11(n)) -> MLP (2,4_NL,1_L)/23(Wx_11(n))
  BK (2,4_NL,1_L)/6(Wx_10(n)) -> MLP (2,4_NL,1_L)/24(Wx_10(n))
  BK (2,4_NL,1_L)/5(Wy_14(n)) -> MLP (2,4_NL,1_L)/25(Wy_14(n))
  BK (2,4_NL,1_L)/4(Wy_13(n)) -> MLP (2,4_NL,1_L)/26(Wy_13(n))
  BK (2,4_NL,1_L)/3(Wy_12(n)) -> MLP (2,4_NL,1_L)/27(Wy_12(n))
  x_4(n)/1 -> MLP (2,4_NL,1_L)/1(x_4(n))
  x_3(n)/1 -> MLP (2,4_NL,1_L)/2(x_3(n))
  x_2(n)/1 -> MLP (2,4_NL,1_L)/3(x_2(n))
  BK (2,4_NL,1_L)/2(Wy_11(n)) -> MLP (2,4_NL,1_L)/28(Wy_11(n))
  AddSub/1 -> BK (2,4_NL,1_L)/11(e(n)), e(n)/1
  BK (2,4_NL,1_L)/1(Wy_10(n)) -> MLP (2,4_NL,1_L)/29(Wy_10(n))
  x_1(n)/1 -> MLP (2,4_NL,1_L)/4(x_1(n))
  y_ref(n)/1 -> Delay/1
  Delay/1 -> AddSub/1

== system Relu_NoOutFB_4_4_1_HW_C6/EN_MLP_BK_(1,4_NL,1_L)_HW_FPGA4/MLP_BK_(2,4_NL,1_L)_HW_FPGA ==
  x_1(n) : Inport
  x_2(n) : Inport  Port=2
  x_3(n) : Inport  Port=3
  x_4(n) : Inport  Port=4
  y_ref(n) : Inport  Port=5
  AddSub : xbsIndex_r4/AddSub  mode=Subtraction  use_carryin=off  use_carryout=off  en=off  latency=0  precision=User Defined  arith_type="Signed  (2's comp)"  n_bits=nb  bin_pt=bp  quantization="Round  (unbiased: +/- Inf)"  overflow=Wrap  dbl_ovrd=off  use_behavioral_HDL=off  hw_selection=Fabric  pipelined=off  block_type=addsub
  BK (2,4_NL,1_L) : Subsystem
  Delay{,1..4} (5 alike) : xbsIndex_r4/Delay  rst=off  infoeditControl=Selection of Reset will increase slice count due to use of real FFs and instead of SRLs  en=off  latency=delayROMSig+delayMulx+delayMuly  dbl_ovrd=off  reg_retiming=off  block_type=delay
  MLP (2,4_NL,1_L) : Subsystem
  y(n) : Outport
  e(n) : Outport  Port=2
  wires:
  Delay/1 -> AddSub/1
  y_ref(n)/1 -> Delay/1
  x_1(n)/1 -> MLP (2,4_NL,1_L)/4(x_1(n))
  BK (2,4_NL,1_L)/1(Wy_10(n)) -> MLP (2,4_NL,1_L)/29(Wy_10(n))
  AddSub/1 -> e(n)/1, BK (2,4_NL,1_L)/11(e(n))
  BK (2,4_NL,1_L)/2(Wy_11(n)) -> MLP (2,4_NL,1_L)/28(Wy_11(n))
  x_2(n)/1 -> MLP (2,4_NL,1_L)/3(x_2(n))
  x_3(n)/1 -> MLP (2,4_NL,1_L)/2(x_3(n))
  x_4(n)/1 -> MLP (2,4_NL,1_L)/1(x_4(n))
  BK (2,4_NL,1_L)/3(Wy_12(n)) -> MLP (2,4_NL,1_L)/27(Wy_12(n))
  BK (2,4_NL,1_L)/4(Wy_13(n)) -> MLP (2,4_NL,1_L)/26(Wy_13(n))
  BK (2,4_NL,1_L)/5(Wy_14(n)) -> MLP (2,4_NL,1_L)/25(Wy_14(n))
  BK (2,4_NL,1_L)/6(Wx_10(n)) -> MLP (2,4_NL,1_L)/24(Wx_10(n))
  BK (2,4_NL,1_L)/7(Wx_11(n)) -> MLP (2,4_NL,1_L)/23(Wx_11(n))
  BK (2,4_NL,1_L)/8(Wx_12(n)) -> MLP (2,4_NL,1_L)/22(Wx_12(n))
  BK (2,4_NL,1_L)/9(Wx_13(n)) -> MLP (2,4_NL,1_L)/21(Wx_13(n))
  BK (2,4_NL,1_L)/10(Wx_14(n)) -> MLP (2,4_NL,1_L)/20(Wx_14(n))
  BK (2,4_NL,1_L)/11(Wx_20(n)) -> MLP (2,4_NL,1_L)/19(Wx_20(n))
  BK (2,4_NL,1_L)/12(Wx_21(n)) -> MLP (2,4_NL,1_L)/18(Wx_21(n))
  BK (2,4_NL,1_L)/13(Wx_22(n)) -> MLP (2,4_NL,1_L)/17(Wx_22(n))
  BK (2,4_NL,1_L)/14(Wx_23(n)) -> MLP (2,4_NL,1_L)/16(Wx_23(n))
  BK (2,4_NL,1_L)/15(Wx_24(n)) -> MLP (2,4_NL,1_L)/15(Wx_24(n))
  BK (2,4_NL,1_L)/16(Wx_30(n)) -> MLP (2,4_NL,1_L)/14(Wx_30(n))
  BK (2,4_NL,1_L)/17(Wx_31(n)) -> MLP (2,4_NL,1_L)/13(Wx_31(n))
  BK (2,4_NL,1_L)/18(Wx_32(n)) -> MLP (2,4_NL,1_L)/12(Wx_32(n)1)
  BK (2,4_NL,1_L)/19(Wx_33(n)) -> MLP (2,4_NL,1_L)/11(Wx_33(n))
  BK (2,4_NL,1_L)/20(Wx_34(n)) -> MLP (2,4_NL,1_L)/10(Wx_34(n))
  BK (2,4_NL,1_L)/21(Wx_40(n)) -> MLP (2,4_NL,1_L)/9(Wx_40(n))
  BK (2,4_NL,1_L)/22(Wx_41(n)) -> MLP (2,4_NL,1_L)/8(Wx_41(n))
  BK (2,4_NL,1_L)/23(Wx_42(n)) -> MLP (2,4_NL,1_L)/7(Wx_42(n))
  BK (2,4_NL,1_L)/24(Wx_43(n)) -> MLP (2,4_NL,1_L)/6(Wx_43(n))
  BK (2,4_NL,1_L)/25(Wx_44(n)) -> MLP (2,4_NL,1_L)/5(Wx_44(n))
  MLP (2,4_NL,1_L)/11(x_4(n)bp) -> Delay1/1
  MLP (2,4_NL,1_L)/10(x_3(n)bp) -> Delay2/1
  MLP (2,4_NL,1_L)/9(x_2(n)bp) -> Delay3/1
  MLP (2,4_NL,1_L)/8(x_1(n)bp) -> Delay4/1
  MLP (2,4_NL,1_L)/6(z_4(n)) -> BK (2,4_NL,1_L)/6(z_4(n))
  MLP (2,4_NL,1_L)/5(z_3(n)) -> BK (2,4_NL,1_L)/7(z_3(n))
  MLP (2,4_NL,1_L)/4(z_2(n)) -> BK (2,4_NL,1_L)/8(z_2(n))
  MLP (2,4_NL,1_L)/3(z_1(n)) -> BK (2,4_NL,1_L)/9(z_1(n))
  MLP (2,4_NL,1_L)/2(z_0(n)) -> BK (2,4_NL,1_L)/10(z_0(n))
  MLP (2,4_NL,1_L)/1(y_0(n)) -> y(n)/1, AddSub/2
  Delay1/1 -> BK (2,4_NL,1_L)/1(x_4(n))
  Delay2/1 -> BK (2,4_NL,1_L)/2(x_3(n))
  Delay3/1 -> BK (2,4_NL,1_L)/3(x_2(n))
  Delay4/1 -> BK (2,4_NL,1_L)/4(x_1(n))
  MLP (2,4_NL,1_L)/7(x_0(n)bp) -> BK (2,4_NL,1_L)/5(x_0(n))

== system Relu_NoOutFB_4_4_1_HW_C6/EN_MLP_BK_(1,4_NL,1_L)_HW_FPGA5/MLP_BK_(2,4_NL,1_L)_HW_FPGA ==
  x_1(n) : Inport
  x_2(n) : Inport  Port=2
  x_3(n) : Inport  Port=3
  x_4(n) : Inport  Port=4
  y_ref(n) : Inport  Port=5
  AddSub : xbsIndex_r4/AddSub  mode=Subtraction  use_carryin=off  use_carryout=off  en=off  latency=0  precision=User Defined  arith_type="Signed  (2's comp)"  n_bits=nb  bin_pt=bp  quantization="Round  (unbiased: +/- Inf)"  overflow=Wrap  dbl_ovrd=off  use_behavioral_HDL=off  hw_selection=Fabric  pipelined=off  block_type=addsub
  BK (2,4_NL,1_L) : Subsystem
  Delay{,1..4} (5 alike) : xbsIndex_r4/Delay  rst=off  infoeditControl=Selection of Reset will increase slice count due to use of real FFs and instead of SRLs  en=off  latency=delayROMSig+delayMulx+delayMuly  dbl_ovrd=off  reg_retiming=off  block_type=delay
  MLP (2,4_NL,1_L) : Subsystem
  y(n) : Outport
  e(n) : Outport  Port=2
  wires:
  MLP (2,4_NL,1_L)/7(x_0(n)bp) -> BK (2,4_NL,1_L)/5(x_0(n))
  Delay4/1 -> BK (2,4_NL,1_L)/4(x_1(n))
  Delay3/1 -> BK (2,4_NL,1_L)/3(x_2(n))
  Delay2/1 -> BK (2,4_NL,1_L)/2(x_3(n))
  Delay1/1 -> BK (2,4_NL,1_L)/1(x_4(n))
  MLP (2,4_NL,1_L)/1(y_0(n)) -> AddSub/2, y(n)/1
  MLP (2,4_NL,1_L)/2(z_0(n)) -> BK (2,4_NL,1_L)/10(z_0(n))
  MLP (2,4_NL,1_L)/3(z_1(n)) -> BK (2,4_NL,1_L)/9(z_1(n))
  MLP (2,4_NL,1_L)/4(z_2(n)) -> BK (2,4_NL,1_L)/8(z_2(n))
  MLP (2,4_NL,1_L)/5(z_3(n)) -> BK (2,4_NL,1_L)/7(z_3(n))
  MLP (2,4_NL,1_L)/6(z_4(n)) -> BK (2,4_NL,1_L)/6(z_4(n))
  MLP (2,4_NL,1_L)/8(x_1(n)bp) -> Delay4/1
  MLP (2,4_NL,1_L)/9(x_2(n)bp) -> Delay3/1
  MLP (2,4_NL,1_L)/10(x_3(n)bp) -> Delay2/1
  MLP (2,4_NL,1_L)/11(x_4(n)bp) -> Delay1/1
  BK (2,4_NL,1_L)/25(Wx_44(n)) -> MLP (2,4_NL,1_L)/5(Wx_44(n))
  BK (2,4_NL,1_L)/24(Wx_43(n)) -> MLP (2,4_NL,1_L)/6(Wx_43(n))
  BK (2,4_NL,1_L)/23(Wx_42(n)) -> MLP (2,4_NL,1_L)/7(Wx_42(n))
  BK (2,4_NL,1_L)/22(Wx_41(n)) -> MLP (2,4_NL,1_L)/8(Wx_41(n))
  BK (2,4_NL,1_L)/21(Wx_40(n)) -> MLP (2,4_NL,1_L)/9(Wx_40(n))
  BK (2,4_NL,1_L)/20(Wx_34(n)) -> MLP (2,4_NL,1_L)/10(Wx_34(n))
  BK (2,4_NL,1_L)/19(Wx_33(n)) -> MLP (2,4_NL,1_L)/11(Wx_33(n))
  BK (2,4_NL,1_L)/18(Wx_32(n)) -> MLP (2,4_NL,1_L)/12(Wx_32(n)1)
  BK (2,4_NL,1_L)/17(Wx_31(n)) -> MLP (2,4_NL,1_L)/13(Wx_31(n))
  BK (2,4_NL,1_L)/16(Wx_30(n)) -> MLP (2,4_NL,1_L)/14(Wx_30(n))
  BK (2,4_NL,1_L)/15(Wx_24(n)) -> MLP (2,4_NL,1_L)/15(Wx_24(n))
  BK (2,4_NL,1_L)/14(Wx_23(n)) -> MLP (2,4_NL,1_L)/16(Wx_23(n))
  BK (2,4_NL,1_L)/13(Wx_22(n)) -> MLP (2,4_NL,1_L)/17(Wx_22(n))
  BK (2,4_NL,1_L)/12(Wx_21(n)) -> MLP (2,4_NL,1_L)/18(Wx_21(n))
  BK (2,4_NL,1_L)/11(Wx_20(n)) -> MLP (2,4_NL,1_L)/19(Wx_20(n))
  BK (2,4_NL,1_L)/10(Wx_14(n)) -> MLP (2,4_NL,1_L)/20(Wx_14(n))
  BK (2,4_NL,1_L)/9(Wx_13(n)) -> MLP (2,4_NL,1_L)/21(Wx_13(n))
  BK (2,4_NL,1_L)/8(Wx_12(n)) -> MLP (2,4_NL,1_L)/22(Wx_12(n))
  BK (2,4_NL,1_L)/7(Wx_11(n)) -> MLP (2,4_NL,1_L)/23(Wx_11(n))
  BK (2,4_NL,1_L)/6(Wx_10(n)) -> MLP (2,4_NL,1_L)/24(Wx_10(n))
  BK (2,4_NL,1_L)/5(Wy_14(n)) -> MLP (2,4_NL,1_L)/25(Wy_14(n))
  BK (2,4_NL,1_L)/4(Wy_13(n)) -> MLP (2,4_NL,1_L)/26(Wy_13(n))
  BK (2,4_NL,1_L)/3(Wy_12(n)) -> MLP (2,4_NL,1_L)/27(Wy_12(n))
  x_4(n)/1 -> MLP (2,4_NL,1_L)/1(x_4(n))
  x_3(n)/1 -> MLP (2,4_NL,1_L)/2(x_3(n))
  x_2(n)/1 -> MLP (2,4_NL,1_L)/3(x_2(n))
  BK (2,4_NL,1_L)/2(Wy_11(n)) -> MLP (2,4_NL,1_L)/28(Wy_11(n))
  AddSub/1 -> BK (2,4_NL,1_L)/11(e(n)), e(n)/1
  BK (2,4_NL,1_L)/1(Wy_10(n)) -> MLP (2,4_NL,1_L)/29(Wy_10(n))
  x_1(n)/1 -> MLP (2,4_NL,1_L)/4(x_1(n))
  y_ref(n)/1 -> Delay/1
  Delay/1 -> AddSub/1

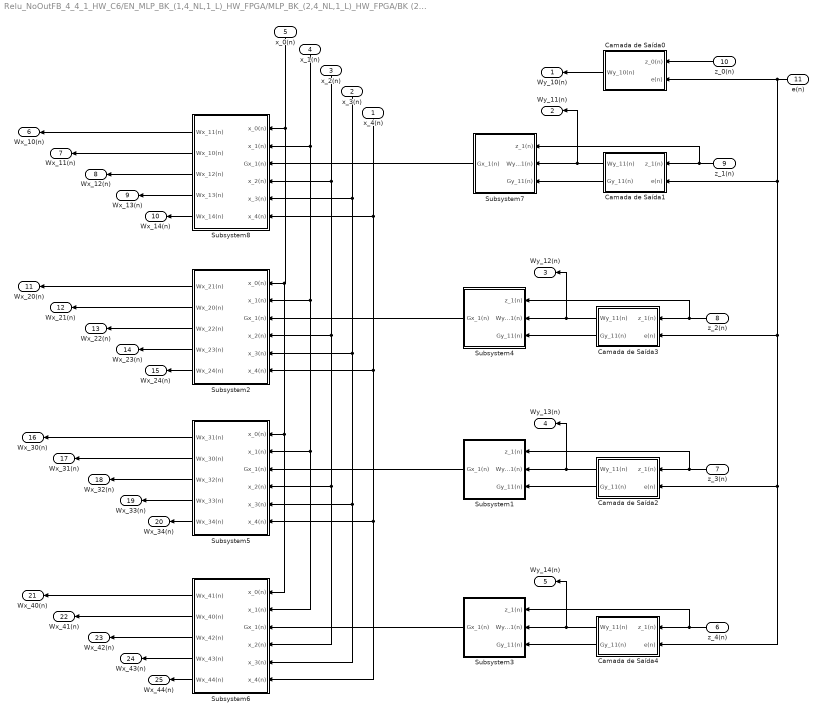
== system Relu_NoOutFB_4_4_1_HW_C6/EN_MLP_BK_(1,4_NL,1_L)_HW_FPGA/MLP_BK_(2,4_NL,1_L)_HW_FPGA/BK (2,4_NL,1_L) ==
  x_4(n) : Inport
  x_3(n) : Inport  Port=2
  x_2(n) : Inport  Port=3
  x_1(n) : Inport  Port=4
  x_0(n) : Inport  Port=5
  z_4(n) : Inport  Port=6
  z_3(n) : Inport  Port=7
  z_2(n) : Inport  Port=8
  z_1(n) : Inport  Port=9
  z_0(n) : Inport  Port=10
  e(n) : Inport  Port=11
  Camada de Saída0 : Subsystem
  Camada de Saída1 : Subsystem
  Camada de Saída2 : Subsystem
  Camada de Saída3 : Subsystem
  Camada de Saída4 : Subsystem
  Subsystem1 : Subsystem
  Subsystem2 : Subsystem
  Subsystem3 : Subsystem
  Subsystem4 : Subsystem
  Subsystem5 : Subsystem
  Subsystem6 : Subsystem
  Subsystem7 : Subsystem
  Subsystem8 : Subsystem
  Wy_10(n) : Outport
  Wy_11(n) : Outport  Port=2
  Wy_12(n) : Outport  Port=3
  Wy_13(n) : Outport  Port=4
  Wy_14(n) : Outport  Port=5
  Wx_10(n) : Outport  Port=6
  Wx_11(n) : Outport  Port=7
  Wx_12(n) : Outport  Port=8
  Wx_13(n) : Outport  Port=9
  Wx_14(n) : Outport  Port=10
  Wx_20(n) : Outport  Port=11
  Wx_21(n) : Outport  Port=12
  Wx_22(n) : Outport  Port=13
  Wx_23(n) : Outport  Port=14
  Wx_24(n) : Outport  Port=15
  Wx_30(n) : Outport  Port=16
  Wx_31(n) : Outport  Port=17
  Wx_32(n) : Outport  Port=18
  Wx_33(n) : Outport  Port=19
  Wx_34(n) : Outport  Port=20
  Wx_40(n) : Outport  Port=21
  Wx_41(n) : Outport  Port=22
  Wx_42(n) : Outport  Port=23
  Wx_43(n) : Outport  Port=24
  Wx_44(n) : Outport  Port=25
  wires:
  e(n)/1 -> Camada de Saída0/2(e(n)), Camada de Saída1/2(e(n)), Camada de Saída4/2(e(n)), Camada de Saída2/2(e(n)), Camada de Saída3/2(e(n))
  Camada de Saída0/1(Wy_10(n)) -> Wy_10(n)/1
  z_1(n)/1 -> Subsystem7/1(z_1(n)), Camada de Saída1/1(z_1(n))
  z_0(n)/1 -> Camada de Saída0/1(z_0(n))
  Camada de Saída1/2(Gy_11(n)) -> Subsystem7/3(Gy_11(n))
  Camada de Saída1/1(Wy_11(n)) -> Subsystem7/2(Wy_11(n)), Wy_11(n)/1
  Subsystem7/1(Gx_1(n)) -> Subsystem8/3(Gx_1(n))
  Subsystem8/1(Wx_11(n)) -> Wx_10(n)/1
  Subsystem8/2(Wx_10(n)) -> Wx_11(n)/1
  z_2(n)/1 -> Subsystem4/1(z_1(n)), Camada de Saída3/1(z_1(n))
  Camada de Saída3/2(Gy_11(n)) -> Subsystem4/3(Gy_11(n))
  Camada de Saída3/1(Wy_11(n)) -> Subsystem4/2(Wy_11(n)), Wy_12(n)/1
  z_3(n)/1 -> Subsystem1/1(z_1(n)), Camada de Saída2/1(z_1(n))
  Camada de Saída2/2(Gy_11(n)) -> Subsystem1/3(Gy_11(n))
  Camada de Saída2/1(Wy_11(n)) -> Subsystem1/2(Wy_11(n)), Wy_13(n)/1
  z_4(n)/1 -> Subsystem3/1(z_1(n)), Camada de Saída4/1(z_1(n))
  Camada de Saída4/2(Gy_11(n)) -> Subsystem3/3(Gy_11(n))
  Camada de Saída4/1(Wy_11(n)) -> Subsystem3/2(Wy_11(n)), Wy_14(n)/1
  Subsystem3/1(Gx_1(n)) -> Subsystem6/3(Gx_1(n))
  Subsystem8/3(Wx_12(n)) -> Wx_12(n)/1
  Subsystem8/4(Wx_13(n)) -> Wx_13(n)/1
  Subsystem8/5(Wx_14(n)) -> Wx_14(n)/1
  Subsystem4/1(Gx_1(n)) -> Subsystem2/3(Gx_1(n))
  x_1(n)/1 -> Subsystem8/2(x_1(n)), Subsystem2/2(x_1(n)), Subsystem6/2(x_1(n)), Subsystem5/2(x_1(n))
  x_0(n)/1 -> Subsystem8/1(x_0(n)), Subsystem2/1(x_0(n)), Subsystem6/1(x_0(n)), Subsystem5/1(x_0(n))
  x_3(n)/1 -> Subsystem8/5(x_3(n)), Subsystem2/5(x_3(n)), Subsystem6/5(x_3(n)), Subsystem5/5(x_3(n))
  x_2(n)/1 -> Subsystem8/4(x_2(n)), Subsystem2/4(x_2(n)), Subsystem6/4(x_2(n)), Subsystem5/4(x_2(n))
  x_4(n)/1 -> Subsystem8/6(x_4(n)), Subsystem2/6(x_4(n)), Subsystem6/6(x_4(n)), Subsystem5/6(x_4(n))
  Subsystem1/1(Gx_1(n)) -> Subsystem5/3(Gx_1(n))
  Subsystem2/1(Wx_21(n)) -> Wx_20(n)/1
  Subsystem2/2(Wx_20(n)) -> Wx_21(n)/1
  Subsystem2/3(Wx_22(n)) -> Wx_22(n)/1
  Subsystem2/4(Wx_23(n)) -> Wx_23(n)/1
  Subsystem2/5(Wx_24(n)) -> Wx_24(n)/1
  Subsystem5/1(Wx_31(n)) -> Wx_30(n)/1
  Subsystem5/2(Wx_30(n)) -> Wx_31(n)/1
  Subsystem5/3(Wx_32(n)) -> Wx_32(n)/1
  Subsystem5/4(Wx_33(n)) -> Wx_33(n)/1
  Subsystem5/5(Wx_34(n)) -> Wx_34(n)/1
  Subsystem6/1(Wx_41(n)) -> Wx_40(n)/1
  Subsystem6/2(Wx_40(n)) -> Wx_41(n)/1
  Subsystem6/3(Wx_42(n)) -> Wx_42(n)/1
  Subsystem6/4(Wx_43(n)) -> Wx_43(n)/1
  Subsystem6/5(Wx_44(n)) -> Wx_44(n)/1

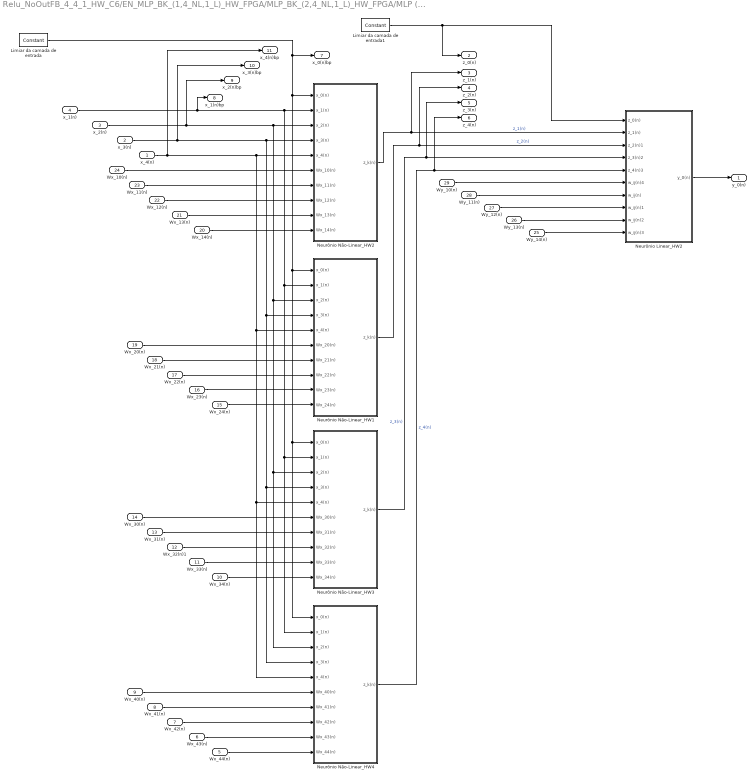
== system Relu_NoOutFB_4_4_1_HW_C6/EN_MLP_BK_(1,4_NL,1_L)_HW_FPGA/MLP_BK_(2,4_NL,1_L)_HW_FPGA/MLP (2,4_NL,1_L) ==
  x_4(n) : Inport
  x_3(n) : Inport  Port=2
  x_2(n) : Inport  Port=3
  x_1(n) : Inport  Port=4
  Wx_44(n) : Inport  Port=5
  Wx_43(n) : Inport  Port=6
  Wx_42(n) : Inport  Port=7
  Wx_41(n) : Inport  Port=8
  Wx_40(n) : Inport  Port=9
  Wx_34(n) : Inport  Port=10
  Wx_33(n) : Inport  Port=11
  Wx_32(n)1 : Inport  Port=12
  Wx_31(n) : Inport  Port=13
  Wx_30(n) : Inport  Port=14
  Wx_24(n) : Inport  Port=15
  Wx_23(n) : Inport  Port=16
  Wx_22(n) : Inport  Port=17
  Wx_21(n) : Inport  Port=18
  Wx_20(n) : Inport  Port=19
  Wx_14(n) : Inport  Port=20
  Wx_13(n) : Inport  Port=21
  Wx_12(n) : Inport  Port=22
  Wx_11(n) : Inport  Port=23
  Wx_10(n) : Inport  Port=24
  Wy_14(n) : Inport  Port=25
  Wy_13(n) : Inport  Port=26
  Wy_12(n) : Inport  Port=27
  Wy_11(n) : Inport  Port=28
  Wy_10(n) : Inport  Port=29
  Limiar da camada de entrada : xbsIndex_r4/Constant  const=1  gui_display_data_type=Fixed-point  arith_type=Signed (2's comp)  n_bits=nb  bin_pt=bp  preci_type=Single  exp_width=8  frac_width=24  explicit_period=off  period=0.01  equ=P=C  opselect=C  inp2=PCIN>>17  opr=+  inp1=P  carry=CIN  dbl_ovrd=off  block_type=constant
  Limiar da camada de entrada1 : xbsIndex_r4/Constant  const=1  gui_display_data_type=Fixed-point  arith_type=Signed (2's comp)  n_bits=nb  bin_pt=bp  preci_type=Single  exp_width=8  frac_width=24  explicit_period=off  period=0.01  equ=P=C  opselect=C  inp2=PCIN>>17  opr=+  inp1=P  carry=CIN  dbl_ovrd=off  block_type=constant
  Neurônio Linear_HW2 : Subsystem
  Neurônio Não-Linear_HW1 : Subsystem
  Neurônio Não-Linear_HW2 : Subsystem
  Neurônio Não-Linear_HW3 : Subsystem
  Neurônio Não-Linear_HW4 : Subsystem
  y_0(n) : Outport
  z_0(n) : Outport  Port=2
  z_1(n) : Outport  Port=3
  z_2(n) : Outport  Port=4
  z_3(n) : Outport  Port=5
  z_4(n) : Outport  Port=6
  x_0(n)bp : Outport  Port=7
  x_1(n)bp : Outport  Port=8
  x_2(n)bp : Outport  Port=9
  x_3(n)bp : Outport  Port=10
  x_4(n)bp : Outport  Port=11
  wires:
  Wy_14(n)/1 -> Neurônio Linear_HW2/10(w_ij(n)3)
  Wy_13(n)/1 -> Neurônio Linear_HW2/9(w_ij(n)2)
  Wy_12(n)/1 -> Neurônio Linear_HW2/8(w_ij(n)1)
  Wy_11(n)/1 -> Neurônio Linear_HW2/7(w_ij(n))
  Wy_10(n)/1 -> Neurônio Linear_HW2/6(w_ij(n)4)
  Wx_41(n)/1 -> Neurônio Não-Linear_HW4/7(Wx_41(n))
  Wx_40(n)/1 -> Neurônio Não-Linear_HW4/6(Wx_40(n))
  Limiar da camada de entrada/1 -> Neurônio Não-Linear_HW2/1(x_0(n)), Neurônio Não-Linear_HW4/1(x_0(n)), Neurônio Não-Linear_HW3/1(x_0(n)), Neurônio Não-Linear_HW1/1(x_0(n)), x_0(n)bp/1
  Neurônio Não-Linear_HW4/1(z_k(n)) -> Neurônio Linear_HW2/5(z_4(n)3), z_4(n)/1  "z_4(n)"
  Neurônio Não-Linear_HW3/1(z_k(n)) -> Neurônio Linear_HW2/4(z_3(n)2), z_3(n)/1  "z_3(n)"
  Neurônio Não-Linear_HW2/1(z_k(n)) -> Neurônio Linear_HW2/2(z_1(n)), z_1(n)/1  "z_1(n)"
  Neurônio Linear_HW2/1(y_0(n)) -> y_0(n)/1
  Neurônio Não-Linear_HW1/1(z_k(n)) -> Neurônio Linear_HW2/3(z_2(n)1), z_2(n)/1  "z_2(n)"
  Wx_43(n)/1 -> Neurônio Não-Linear_HW4/9(Wx_43(n))
  Wx_42(n)/1 -> Neurônio Não-Linear_HW4/8(Wx_42(n))
  Wx_44(n)/1 -> Neurônio Não-Linear_HW4/10(Wx_44(n))
  Wx_31(n)/1 -> Neurônio Não-Linear_HW3/7(Wx_31(n))
  Wx_30(n)/1 -> Neurônio Não-Linear_HW3/6(Wx_30(n))
  Wx_33(n)/1 -> Neurônio Não-Linear_HW3/9(Wx_33(n))
  Wx_32(n)1/1 -> Neurônio Não-Linear_HW3/8(Wx_32(n))
  Wx_34(n)/1 -> Neurônio Não-Linear_HW3/10(Wx_34(n))
  Wx_21(n)/1 -> Neurônio Não-Linear_HW1/7(Wx_21(n))
  Wx_20(n)/1 -> Neurônio Não-Linear_HW1/6(Wx_20(n))
  Wx_23(n)/1 -> Neurônio Não-Linear_HW1/9(Wx_23(n))
  Wx_22(n)/1 -> Neurônio Não-Linear_HW1/8(Wx_22(n))
  Wx_24(n)/1 -> Neurônio Não-Linear_HW1/10(Wx_24(n))
  Wx_11(n)/1 -> Neurônio Não-Linear_HW2/7(Wx_11(n))
  Wx_10(n)/1 -> Neurônio Não-Linear_HW2/6(Wx_10(n))
  Wx_13(n)/1 -> Neurônio Não-Linear_HW2/9(Wx_13(n))
  Wx_12(n)/1 -> Neurônio Não-Linear_HW2/8(Wx_12(n))
  Wx_14(n)/1 -> Neurônio Não-Linear_HW2/10(Wx_14(n))
  x_1(n)/1 -> Neurônio Não-Linear_HW2/2(x_1(n)), Neurônio Não-Linear_HW4/2(x_1(n)), Neurônio Não-Linear_HW3/2(x_1(n)), Neurônio Não-Linear_HW1/2(x_1(n)), x_1(n)bp/1
  x_2(n)/1 -> Neurônio Não-Linear_HW4/3(x_2(n)), Neurônio Não-Linear_HW3/3(x_2(n)), Neurônio Não-Linear_HW1/3(x_2(n)), Neurônio Não-Linear_HW2/3(x_2(n)), x_2(n)bp/1
  x_3(n)/1 -> x_3(n)bp/1, Neurônio Não-Linear_HW4/4(x_3(n)), Neurônio Não-Linear_HW3/4(x_3(n)), Neurônio Não-Linear_HW1/4(x_3(n)), Neurônio Não-Linear_HW2/4(x_3(n))
  x_4(n)/1 -> x_4(n)bp/1, Neurônio Não-Linear_HW4/5(x_4(n)), Neurônio Não-Linear_HW3/5(x_4(n)), Neurônio Não-Linear_HW1/5(x_4(n)), Neurônio Não-Linear_HW2/5(x_4(n))
  Limiar da camada de entrada1/1 -> Neurônio Linear_HW2/1(z_0(n)), z_0(n)/1

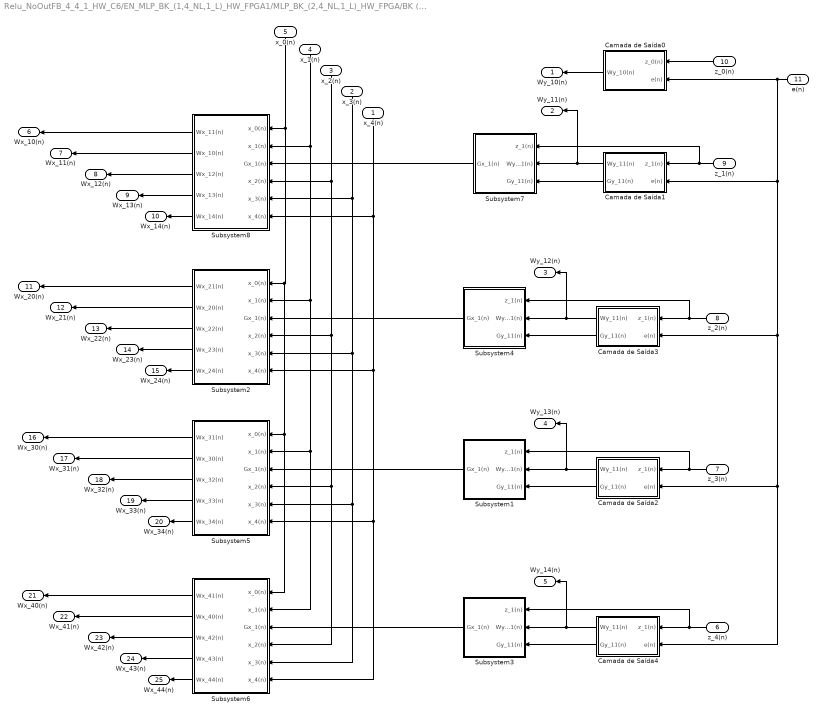
== system Relu_NoOutFB_4_4_1_HW_C6/EN_MLP_BK_(1,4_NL,1_L)_HW_FPGA1/MLP_BK_(2,4_NL,1_L)_HW_FPGA/BK (2,4_NL,1_L) ==
  x_4(n) : Inport
  x_3(n) : Inport  Port=2
  x_2(n) : Inport  Port=3
  x_1(n) : Inport  Port=4
  x_0(n) : Inport  Port=5
  z_4(n) : Inport  Port=6
  z_3(n) : Inport  Port=7
  z_2(n) : Inport  Port=8
  z_1(n) : Inport  Port=9
  z_0(n) : Inport  Port=10
  e(n) : Inport  Port=11
  Camada de Saída0 : Subsystem
  Camada de Saída1 : Subsystem
  Camada de Saída2 : Subsystem
  Camada de Saída3 : Subsystem
  Camada de Saída4 : Subsystem
  Subsystem1 : Subsystem
  Subsystem2 : Subsystem
  Subsystem3 : Subsystem
  Subsystem4 : Subsystem
  Subsystem5 : Subsystem
  Subsystem6 : Subsystem
  Subsystem7 : Subsystem
  Subsystem8 : Subsystem
  Wy_10(n) : Outport
  Wy_11(n) : Outport  Port=2
  Wy_12(n) : Outport  Port=3
  Wy_13(n) : Outport  Port=4
  Wy_14(n) : Outport  Port=5
  Wx_10(n) : Outport  Port=6
  Wx_11(n) : Outport  Port=7
  Wx_12(n) : Outport  Port=8
  Wx_13(n) : Outport  Port=9
  Wx_14(n) : Outport  Port=10
  Wx_20(n) : Outport  Port=11
  Wx_21(n) : Outport  Port=12
  Wx_22(n) : Outport  Port=13
  Wx_23(n) : Outport  Port=14
  Wx_24(n) : Outport  Port=15
  Wx_30(n) : Outport  Port=16
  Wx_31(n) : Outport  Port=17
  Wx_32(n) : Outport  Port=18
  Wx_33(n) : Outport  Port=19
  Wx_34(n) : Outport  Port=20
  Wx_40(n) : Outport  Port=21
  Wx_41(n) : Outport  Port=22
  Wx_42(n) : Outport  Port=23
  Wx_43(n) : Outport  Port=24
  Wx_44(n) : Outport  Port=25
  wires:
  Subsystem6/5(Wx_44(n)) -> Wx_44(n)/1
  Subsystem6/4(Wx_43(n)) -> Wx_43(n)/1
  Subsystem6/3(Wx_42(n)) -> Wx_42(n)/1
  Subsystem6/2(Wx_40(n)) -> Wx_41(n)/1
  Subsystem6/1(Wx_41(n)) -> Wx_40(n)/1
  Subsystem5/5(Wx_34(n)) -> Wx_34(n)/1
  Subsystem5/4(Wx_33(n)) -> Wx_33(n)/1
  Subsystem5/3(Wx_32(n)) -> Wx_32(n)/1
  Subsystem5/2(Wx_30(n)) -> Wx_31(n)/1
  Subsystem5/1(Wx_31(n)) -> Wx_30(n)/1
  Subsystem2/5(Wx_24(n)) -> Wx_24(n)/1
  Subsystem2/4(Wx_23(n)) -> Wx_23(n)/1
  Subsystem2/3(Wx_22(n)) -> Wx_22(n)/1
  Subsystem2/2(Wx_20(n)) -> Wx_21(n)/1
  Subsystem2/1(Wx_21(n)) -> Wx_20(n)/1
  Subsystem1/1(Gx_1(n)) -> Subsystem5/3(Gx_1(n))
  x_4(n)/1 -> Subsystem5/6(x_4(n)), Subsystem6/6(x_4(n)), Subsystem2/6(x_4(n)), Subsystem8/6(x_4(n))
  x_2(n)/1 -> Subsystem5/4(x_2(n)), Subsystem6/4(x_2(n)), Subsystem2/4(x_2(n)), Subsystem8/4(x_2(n))
  x_3(n)/1 -> Subsystem5/5(x_3(n)), Subsystem6/5(x_3(n)), Subsystem2/5(x_3(n)), Subsystem8/5(x_3(n))
  x_0(n)/1 -> Subsystem5/1(x_0(n)), Subsystem6/1(x_0(n)), Subsystem2/1(x_0(n)), Subsystem8/1(x_0(n))
  x_1(n)/1 -> Subsystem5/2(x_1(n)), Subsystem6/2(x_1(n)), Subsystem2/2(x_1(n)), Subsystem8/2(x_1(n))
  Subsystem4/1(Gx_1(n)) -> Subsystem2/3(Gx_1(n))
  Subsystem8/5(Wx_14(n)) -> Wx_14(n)/1
  Subsystem8/4(Wx_13(n)) -> Wx_13(n)/1
  Subsystem8/3(Wx_12(n)) -> Wx_12(n)/1
  Subsystem3/1(Gx_1(n)) -> Subsystem6/3(Gx_1(n))
  Camada de Saída4/1(Wy_11(n)) -> Wy_14(n)/1, Subsystem3/2(Wy_11(n))
  Camada de Saída4/2(Gy_11(n)) -> Subsystem3/3(Gy_11(n))
  z_4(n)/1 -> Camada de Saída4/1(z_1(n)), Subsystem3/1(z_1(n))
  Camada de Saída2/1(Wy_11(n)) -> Wy_13(n)/1, Subsystem1/2(Wy_11(n))
  Camada de Saída2/2(Gy_11(n)) -> Subsystem1/3(Gy_11(n))
  z_3(n)/1 -> Camada de Saída2/1(z_1(n)), Subsystem1/1(z_1(n))
  Camada de Saída3/1(Wy_11(n)) -> Wy_12(n)/1, Subsystem4/2(Wy_11(n))
  Camada de Saída3/2(Gy_11(n)) -> Subsystem4/3(Gy_11(n))
  z_2(n)/1 -> Camada de Saída3/1(z_1(n)), Subsystem4/1(z_1(n))
  Subsystem8/2(Wx_10(n)) -> Wx_11(n)/1
  Subsystem8/1(Wx_11(n)) -> Wx_10(n)/1
  Subsystem7/1(Gx_1(n)) -> Subsystem8/3(Gx_1(n))
  Camada de Saída1/1(Wy_11(n)) -> Wy_11(n)/1, Subsystem7/2(Wy_11(n))
  Camada de Saída1/2(Gy_11(n)) -> Subsystem7/3(Gy_11(n))
  z_0(n)/1 -> Camada de Saída0/1(z_0(n))
  z_1(n)/1 -> Camada de Saída1/1(z_1(n)), Subsystem7/1(z_1(n))
  Camada de Saída0/1(Wy_10(n)) -> Wy_10(n)/1
  e(n)/1 -> Camada de Saída3/2(e(n)), Camada de Saída2/2(e(n)), Camada de Saída4/2(e(n)), Camada de Saída1/2(e(n)), Camada de Saída0/2(e(n))

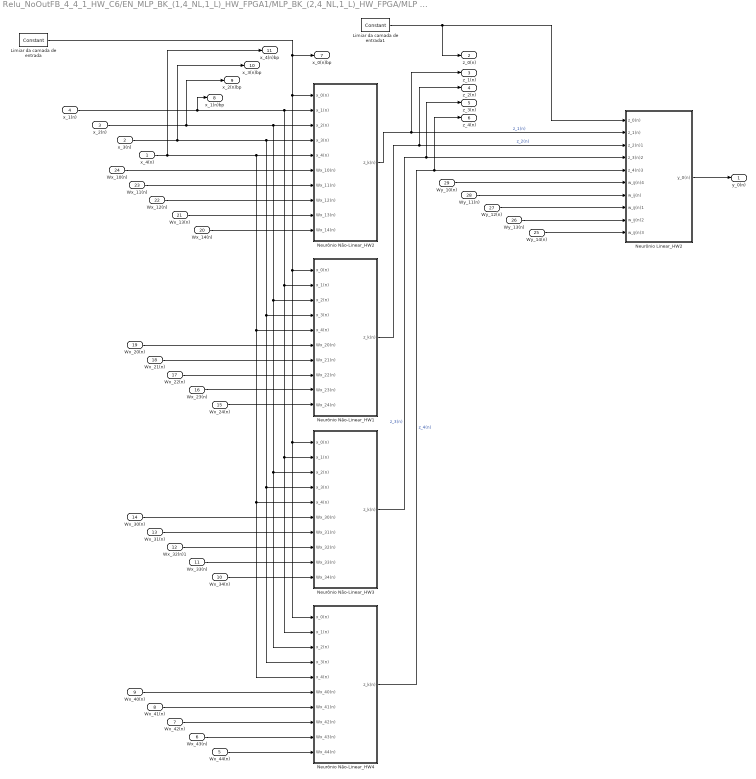
== system Relu_NoOutFB_4_4_1_HW_C6/EN_MLP_BK_(1,4_NL,1_L)_HW_FPGA1/MLP_BK_(2,4_NL,1_L)_HW_FPGA/MLP (2,4_NL,1_L) ==
  x_4(n) : Inport
  x_3(n) : Inport  Port=2
  x_2(n) : Inport  Port=3
  x_1(n) : Inport  Port=4
  Wx_44(n) : Inport  Port=5
  Wx_43(n) : Inport  Port=6
  Wx_42(n) : Inport  Port=7
  Wx_41(n) : Inport  Port=8
  Wx_40(n) : Inport  Port=9
  Wx_34(n) : Inport  Port=10
  Wx_33(n) : Inport  Port=11
  Wx_32(n)1 : Inport  Port=12
  Wx_31(n) : Inport  Port=13
  Wx_30(n) : Inport  Port=14
  Wx_24(n) : Inport  Port=15
  Wx_23(n) : Inport  Port=16
  Wx_22(n) : Inport  Port=17
  Wx_21(n) : Inport  Port=18
  Wx_20(n) : Inport  Port=19
  Wx_14(n) : Inport  Port=20
  Wx_13(n) : Inport  Port=21
  Wx_12(n) : Inport  Port=22
  Wx_11(n) : Inport  Port=23
  Wx_10(n) : Inport  Port=24
  Wy_14(n) : Inport  Port=25
  Wy_13(n) : Inport  Port=26
  Wy_12(n) : Inport  Port=27
  Wy_11(n) : Inport  Port=28
  Wy_10(n) : Inport  Port=29
  Limiar da camada de entrada : xbsIndex_r4/Constant  const=1  gui_display_data_type=Fixed-point  arith_type=Signed (2's comp)  n_bits=nb  bin_pt=bp  preci_type=Single  exp_width=8  frac_width=24  explicit_period=off  period=0.01  equ=P=C  opselect=C  inp2=PCIN>>17  opr=+  inp1=P  carry=CIN  dbl_ovrd=off  block_type=constant
  Limiar da camada de entrada1 : xbsIndex_r4/Constant  const=1  gui_display_data_type=Fixed-point  arith_type=Signed (2's comp)  n_bits=nb  bin_pt=bp  preci_type=Single  exp_width=8  frac_width=24  explicit_period=off  period=0.01  equ=P=C  opselect=C  inp2=PCIN>>17  opr=+  inp1=P  carry=CIN  dbl_ovrd=off  block_type=constant
  Neurônio Linear_HW2 : Subsystem
  Neurônio Não-Linear_HW1 : Subsystem
  Neurônio Não-Linear_HW2 : Subsystem
  Neurônio Não-Linear_HW3 : Subsystem
  Neurônio Não-Linear_HW4 : Subsystem
  y_0(n) : Outport
  z_0(n) : Outport  Port=2
  z_1(n) : Outport  Port=3
  z_2(n) : Outport  Port=4
  z_3(n) : Outport  Port=5
  z_4(n) : Outport  Port=6
  x_0(n)bp : Outport  Port=7
  x_1(n)bp : Outport  Port=8
  x_2(n)bp : Outport  Port=9
  x_3(n)bp : Outport  Port=10
  x_4(n)bp : Outport  Port=11
  wires:
  Limiar da camada de entrada1/1 -> z_0(n)/1, Neurônio Linear_HW2/1(z_0(n))
  x_4(n)/1 -> Neurônio Não-Linear_HW2/5(x_4(n)), Neurônio Não-Linear_HW1/5(x_4(n)), Neurônio Não-Linear_HW3/5(x_4(n)), Neurônio Não-Linear_HW4/5(x_4(n)), x_4(n)bp/1
  x_3(n)/1 -> Neurônio Não-Linear_HW2/4(x_3(n)), Neurônio Não-Linear_HW1/4(x_3(n)), Neurônio Não-Linear_HW3/4(x_3(n)), Neurônio Não-Linear_HW4/4(x_3(n)), x_3(n)bp/1
  x_2(n)/1 -> x_2(n)bp/1, Neurônio Não-Linear_HW2/3(x_2(n)), Neurônio Não-Linear_HW1/3(x_2(n)), Neurônio Não-Linear_HW3/3(x_2(n)), Neurônio Não-Linear_HW4/3(x_2(n))
  x_1(n)/1 -> x_1(n)bp/1, Neurônio Não-Linear_HW1/2(x_1(n)), Neurônio Não-Linear_HW3/2(x_1(n)), Neurônio Não-Linear_HW4/2(x_1(n)), Neurônio Não-Linear_HW2/2(x_1(n))
  Wx_14(n)/1 -> Neurônio Não-Linear_HW2/10(Wx_14(n))
  Wx_12(n)/1 -> Neurônio Não-Linear_HW2/8(Wx_12(n))
  Wx_13(n)/1 -> Neurônio Não-Linear_HW2/9(Wx_13(n))
  Wx_10(n)/1 -> Neurônio Não-Linear_HW2/6(Wx_10(n))
  Wx_11(n)/1 -> Neurônio Não-Linear_HW2/7(Wx_11(n))
  Wx_24(n)/1 -> Neurônio Não-Linear_HW1/10(Wx_24(n))
  Wx_22(n)/1 -> Neurônio Não-Linear_HW1/8(Wx_22(n))
  Wx_23(n)/1 -> Neurônio Não-Linear_HW1/9(Wx_23(n))
  Wx_20(n)/1 -> Neurônio Não-Linear_HW1/6(Wx_20(n))
  Wx_21(n)/1 -> Neurônio Não-Linear_HW1/7(Wx_21(n))
  Wx_34(n)/1 -> Neurônio Não-Linear_HW3/10(Wx_34(n))
  Wx_32(n)1/1 -> Neurônio Não-Linear_HW3/8(Wx_32(n))
  Wx_33(n)/1 -> Neurônio Não-Linear_HW3/9(Wx_33(n))
  Wx_30(n)/1 -> Neurônio Não-Linear_HW3/6(Wx_30(n))
  Wx_31(n)/1 -> Neurônio Não-Linear_HW3/7(Wx_31(n))
  Wx_44(n)/1 -> Neurônio Não-Linear_HW4/10(Wx_44(n))
  Wx_42(n)/1 -> Neurônio Não-Linear_HW4/8(Wx_42(n))
  Wx_43(n)/1 -> Neurônio Não-Linear_HW4/9(Wx_43(n))
  Neurônio Não-Linear_HW1/1(z_k(n)) -> z_2(n)/1, Neurônio Linear_HW2/3(z_2(n)1)  "z_2(n)"
  Neurônio Linear_HW2/1(y_0(n)) -> y_0(n)/1
  Neurônio Não-Linear_HW2/1(z_k(n)) -> z_1(n)/1, Neurônio Linear_HW2/2(z_1(n))  "z_1(n)"
  Neurônio Não-Linear_HW3/1(z_k(n)) -> z_3(n)/1, Neurônio Linear_HW2/4(z_3(n)2)  "z_3(n)"
  Neurônio Não-Linear_HW4/1(z_k(n)) -> z_4(n)/1, Neurônio Linear_HW2/5(z_4(n)3)  "z_4(n)"
  Limiar da camada de entrada/1 -> x_0(n)bp/1, Neurônio Não-Linear_HW1/1(x_0(n)), Neurônio Não-Linear_HW3/1(x_0(n)), Neurônio Não-Linear_HW4/1(x_0(n)), Neurônio Não-Linear_HW2/1(x_0(n))
  Wx_40(n)/1 -> Neurônio Não-Linear_HW4/6(Wx_40(n))
  Wx_41(n)/1 -> Neurônio Não-Linear_HW4/7(Wx_41(n))
  Wy_10(n)/1 -> Neurônio Linear_HW2/6(w_ij(n)4)
  Wy_11(n)/1 -> Neurônio Linear_HW2/7(w_ij(n))
  Wy_12(n)/1 -> Neurônio Linear_HW2/8(w_ij(n)1)
  Wy_13(n)/1 -> Neurônio Linear_HW2/9(w_ij(n)2)
  Wy_14(n)/1 -> Neurônio Linear_HW2/10(w_ij(n)3)
